simulink model "MyEx_3_Nonlinear"  (R2021b)
settings: Solver=VariableStepAuto  StartTime=0.0  StopTime=simTime  RelTol=1e-3
undefined symbols (not defined in the file): b, D, g, k, L, m, MoI, omega, p, p_dot, RPM, TakeStep, Theta
settings Model: Creator=tanzc  LastModifiedBy=tanzc

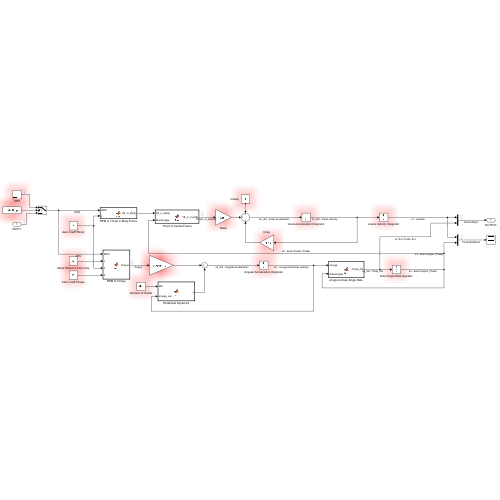
[thumbnail: Simulink's stored preview of the top-level diagram]
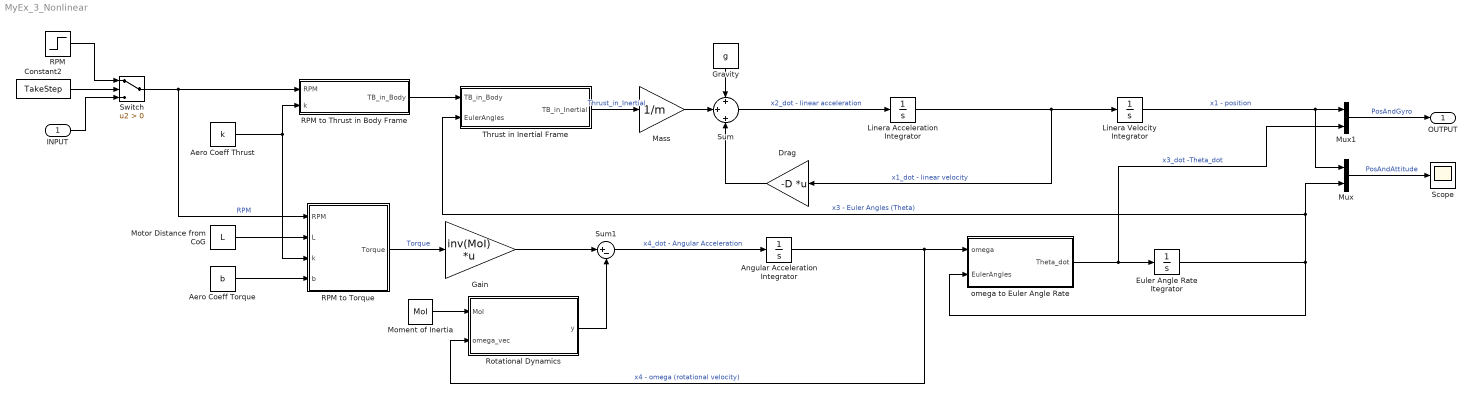
== system MyEx_3_Nonlinear ==
  INPUT : Inport  PortDimensions=4
  Aero Coeff Thrust : Constant  Value=k
  Aero Coeff Torque : Constant  Value=b
  Angular Acceleration Integrator : Integrator  Priority=4  InitialCondition=omega
  Constant2 : Constant  Value=TakeStep
  Drag : Gain  Gain=-D  Multiplication=Matrix(K*u)
  Euler Angle Rate Itegrator : Integrator  Priority=3  InitialCondition=Theta
  Gain : Gain  Gain=inv(MoI)  Multiplication=Matrix(K*u)
  Gravity : Constant  Value=g  VectorParams1D=off
  Linera Acceleration Integrator : Integrator  Priority=2  InitialCondition=p_dot
  Linera Velocity Integrator : Integrator  Priority=1  InitialCondition=p
  Mass : Gain  Gain=1/m
  Moment of Inertia : Constant  Value=MoI  VectorParams1D=off
  Motor Distance from CoG : Constant  Value=L
  Mux : Mux  Inputs=2
  Mux1 : Mux  Inputs=2
  RPM : Step  Time=0  After=RPM  SampleTime=0
  RPM to Thrust in Body Frame : MATLAB Function  TreatAsAtomicUnit=on
  RPM to Torque : MATLAB Function  TreatAsAtomicUnit=on
  Rotational Dynamics : MATLAB Function  TreatAsAtomicUnit=on
  Scope : Scope
  Sum : Sum  Inputs=+|+|+
  Sum1 : Sum  Inputs=|+-
  Switch : Switch  Criteria=u2 > Threshold
  Thrust in Inertial Frame : MATLAB Function  TreatAsAtomicUnit=on
  "omega to Euler Angle Rate " : MATLAB Function  TreatAsAtomicUnit=on
  OUTPUT : Outport
  wires:
  INPUT/1 -> Switch/3
  Mux1/1 -> OUTPUT/1  "PosAndGyro"
  Mux/1 -> Scope/1  "PosAndAttitude"
  RPM to Thrust in Body Frame/1(TB_in_Body) -> Thrust in Inertial Frame/1(TB_in_Body)
  "omega to Euler Angle Rate "/1(Theta_dot) -> Mux1/2, Euler Angle Rate Itegrator/1  "x3_dot -Theta_dot"
  Moment of Inertia/1 -> Rotational Dynamics/1(MoI)
  Switch/1 -> RPM to Thrust in Body Frame/1(RPM), RPM to Torque/1(RPM)  "RPM"
  RPM to Torque/1(Torque) -> Gain/1  "Torque"
  Constant2/1 -> Switch/2
  Aero Coeff Torque/1 -> RPM to Torque/4(b)
  Rotational Dynamics/1(y) -> Sum1/2
  Thrust in Inertial Frame/1(TB_in_Inertial) -> Mass/1  "Thrust_in_Inertial"
  Sum/1 -> Linera Acceleration Integrator/1  "x2_dot - linear acceleration"
  Linera Velocity Integrator/1 -> Mux1/1, Mux/1  "x1 - position"
  Aero Coeff Thrust/1 -> RPM to Thrust in Body Frame/2(k), RPM to Torque/3(k)
  Sum1/1 -> Angular Acceleration Integrator/1  "x4_dot - Angular Acceleration"
  RPM/1 -> Switch/1
  Angular Acceleration Integrator/1 -> "omega to Euler Angle Rate "/1(omega), Rotational Dynamics/2(omega_vec)  "x4 - omega (rotational velocity)"
  Euler Angle Rate Itegrator/1 -> Thrust in Inertial Frame/2(EulerAngles), Mux/2, "omega to Euler Angle Rate "/2(EulerAngles)  "x3 - Euler Angles (Theta)"
  Drag/1 -> Sum/3
  Linera Acceleration Integrator/1 -> Drag/1, Linera Velocity Integrator/1  "x1_dot - linear velocity"
  Gravity/1 -> Sum/1
  Gain/1 -> Sum1/1
  Motor Distance from CoG/1 -> RPM to Torque/2(L)
  Mass/1 -> Sum/2

== matlab function MyEx_3_Nonlinear/RPM to Thrust in Body Frame ==
  data: RPM input; TB_in_Body output; k input
function TB_in_Body = fcn(RPM, k)
TB_in_Body = k * [0; 0; RPM'*RPM];

== matlab function MyEx_3_Nonlinear/Thrust in Inertial Frame ==
  data: TB_in_Body input; EulerAngles input; TB_in_Inertial output
function TB_in_Inertial = fcn(TB_in_Body, EulerAngles)

phi = EulerAngles(1);
theta = EulerAngles(2);
psi = EulerAngles(3);

R = [cos(psi)*cos(theta), cos(psi)*sin(theta)*sin(phi) - sin(psi)*cos(phi), cos(psi)*sin(theta)*cos(phi) + sin(psi)*sin(phi);
    sin(psi)*cos(theta), sin(psi)*sin(theta)*sin(phi) + cos(psi)*cos(phi), sin(psi)*sin(theta)*cos(phi) - cos(psi)*sin(phi);
    -sin(theta), cos(theta)*sin(phi), cos(theta)*cos(phi)];

TB_in_Inertial = R*TB_in_Body;

== matlab function MyEx_3_Nonlinear/RPM to Torque ==
  data: RPM input; Torque output; L input; k input; b input
function Torque = fcn(RPM, L, k, b)

Torque = [  L*k*(RPM(1)^2 - RPM(3)^2); ...
            L*k*(RPM(2)^2 - RPM(4)^2); ...
            b * (RPM(1)^2 - RPM(2)^2 + RPM(3)^2 - RPM(4)^2)];

== matlab function MyEx_3_Nonlinear/Rotational Dynamics ==
  data: MoI input; omega_vec input; y output
function y = fcn(MoI, omega_vec)
Ixx = MoI(1,1);
Iyy = MoI(2,2);
Izz = MoI(3,3);

omega_x = omega_vec(1);
omega_y = omega_vec(2);
omega_z = omega_vec(3);

y = [ (Iyy-Izz)/Ixx*omega_y*omega_z; ...
      (Izz-Ixx)/Iyy*omega_x*omega_z; ...
      (Ixx-Iyy)/Izz*omega_x*omega_y];

== matlab function MyEx_3_Nonlinear/omega to Euler Angle Rate  ==
  data: omega input; Theta_dot output; EulerAngles input
function Theta_dot = fcn(omega, EulerAngles)

phi = EulerAngles(1);
theta = EulerAngles(2);
psi = EulerAngles(3);

B = [ 1, 0, -sin(theta); ...
      0, cos(phi), cos(theta)*sin(phi); ...
      0, -sin(phi), cos(theta)*cos(phi)];
  
Theta_dot = pinv(B)*omega;
